simulink model "fec_ber_hw_V2"  (R2020b)
settings: Solver=FixedStepDiscrete  StartTime=0.0  StopTime=T  RelTol=1e-3
values from neighbouring files (symbols this model uses):
  aximm_awgn_reset = 0    [setup.m]
  aximm_bit_count_reset = 0    [setup.m]
  aximm_bits = n_blocks * k    (= 80)    [setup.m]
  aximm_ctrl_word_dec = 0    [setup.m]
  aximm_ctrl_word_enc = 0    [setup.m]
  aximm_enable = 1    [setup.m]
  aximm_length = k * n_blocks    (= 80)    [setup.m]
  aximm_length_dec = n    (= 160)    [setup.m]
  aximm_length_enc = k    (= 80)    [setup.m]
  aximm_llr_mag_reset = 0    [setup.m]
  aximm_llr_scale = (1/noise_var) * llr_scale    (= 1000)    [setup.m]
  aximm_load_dec = 1    [setup.m]
  aximm_load_enc = 1    [setup.m]
  aximm_noise_std = sqrt(noise_var)    [setup.m]
  aximm_reset = 0    [setup.m]
  d = sqrt(-2*log([0:1/4095:1]))    [setup.m]
  fs = 160e6    (= 160000000)    [setup.m]
  generator_polynomial = '''z^13 + z^12 + z^11 + z^8 + 1'''    [setup.m]
  llr_scale = 7.75/7.75    (= 1)    [setup.m]
libraries: simulink x931, hdlsllib x419, commseqgen3 x52, dspsigops x22, commblkcod2 x3, lib_rfsoc_fec x2
(part 2 of 47)

== system fec_ber_hw_V2/Random Number Generator/Random Number Generator ==
  reset : Inport
  enable : EnablePort
  bit0 : commseqgen3/PN Sequence Generator  poly='z^13 + z^12 + z^11 + z^8 + 1'  ini_sta=[ 1 0 1 0 1 0 1 1 0 1 0 0 1]  outBitMaskSource=Dialog parameter  shift=0  outVarSiz=off  maxOutSizeMode=Dialog parameter  maxOutSize=[10 1]  Ts=-1  sampPerFrame=1  reset=on  bitPackedOutputs=off  outDataType=boolean  numPackedBits=8  bitPackDataSigned=off  bitPackedOutDType=double
  bit1 : commseqgen3/PN Sequence Generator  poly='z^13 + z^12 + z^11 + z^8 + 1'  ini_sta=[ 1 0 0 0 0 0 0 0 0 0 0 1 0]  outBitMaskSource=Dialog parameter  shift=0  outVarSiz=off  maxOutSizeMode=Dialog parameter  maxOutSize=[10 1]  Ts=-1  sampPerFrame=1  reset=on  bitPackedOutputs=off  outDataType=boolean  numPackedBits=8  bitPackDataSigned=off  bitPackedOutDType=double
  bit10 : commseqgen3/PN Sequence Generator  poly='z^13 + z^12 + z^11 + z^8 + 1'  ini_sta=[ 0 0 0 0 0 1 0 1 0 0 0 0 1]  outBitMaskSource=Dialog parameter  shift=0  outVarSiz=off  maxOutSizeMode=Dialog parameter  maxOutSize=[10 1]  Ts=-1  sampPerFrame=1  reset=on  bitPackedOutputs=off  outDataType=boolean  numPackedBits=8  bitPackDataSigned=off  bitPackedOutDType=double
  bit11 : commseqgen3/PN Sequence Generator  poly='z^13 + z^12 + z^11 + z^8 + 1'  ini_sta=[ 0 1 1 0 1 1 1 1 0 1 1 0 1]  outBitMaskSource=Dialog parameter  shift=0  outVarSiz=off  maxOutSizeMode=Dialog parameter  maxOutSize=[10 1]  Ts=-1  sampPerFrame=1  reset=on  bitPackedOutputs=off  outDataType=boolean  numPackedBits=8  bitPackDataSigned=off  bitPackedOutDType=double
  bit12 : commseqgen3/PN Sequence Generator  poly='z^13 + z^12 + z^11 + z^8 + 1'  ini_sta=[ 1 1 0 1 0 1 0 1 0 0 0 0 1]  outBitMaskSource=Dialog parameter  shift=0  outVarSiz=off  maxOutSizeMode=Dialog parameter  maxOutSize=[10 1]  Ts=-1  sampPerFrame=1  reset=on  bitPackedOutputs=off  outDataType=boolean  numPackedBits=8  bitPackDataSigned=off  bitPackedOutDType=double
  bit13 : commseqgen3/PN Sequence Generator  poly='z^13 + z^12 + z^11 + z^8 + 1'  ini_sta=[ 1 0 0 1 1 1 1 0 0 0 0 1 0]  outBitMaskSource=Dialog parameter  shift=0  outVarSiz=off  maxOutSizeMode=Dialog parameter  maxOutSize=[10 1]  Ts=-1  sampPerFrame=1  reset=on  bitPackedOutputs=off  outDataType=boolean  numPackedBits=8  bitPackDataSigned=off  bitPackedOutDType=double
  bit14 : commseqgen3/PN Sequence Generator  poly='z^13 + z^12 + z^11 + z^8 + 1'  ini_sta=[ 1 0 0 0 0 1 0 1 0 0 1 0 1]  outBitMaskSource=Dialog parameter  shift=0  outVarSiz=off  maxOutSizeMode=Dialog parameter  maxOutSize=[10 1]  Ts=-1  sampPerFrame=1  reset=on  bitPackedOutputs=off  outDataType=boolean  numPackedBits=8  bitPackDataSigned=off  bitPackedOutDType=double
  bit15 : commseqgen3/PN Sequence Generator  poly='z^13 + z^12 + z^11 + z^8 + 1'  ini_sta=[ 1 1 0 1 1 1 0 1 0 0 1 0 0]  outBitMaskSource=Dialog parameter  shift=0  outVarSiz=off  maxOutSizeMode=Dialog parameter  maxOutSize=[10 1]  Ts=-1  sampPerFrame=1  reset=on  bitPackedOutputs=off  outDataType=boolean  numPackedBits=8  bitPackDataSigned=off  bitPackedOutDType=double
  bit16 : commseqgen3/PN Sequence Generator  poly='z^13 + z^12 + z^11 + z^8 + 1'  ini_sta=[ 0 0 0 1 1 0 0 1 0 0 0 0 1]  outBitMaskSource=Dialog parameter  shift=0  outVarSiz=off  maxOutSizeMode=Dialog parameter  maxOutSize=[10 1]  Ts=-1  sampPerFrame=1  reset=on  bitPackedOutputs=off  outDataType=boolean  numPackedBits=8  bitPackDataSigned=off  bitPackedOutDType=double
  bit17 : commseqgen3/PN Sequence Generator  poly='z^13 + z^12 + z^11 + z^8 + 1'  ini_sta=[ 1 1 1 0 1 0 0 0 0 1 1 1 0]  outBitMaskSource=Dialog parameter  shift=0  outVarSiz=off  maxOutSizeMode=Dialog parameter  maxOutSize=[10 1]  Ts=-1  sampPerFrame=1  reset=on  bitPackedOutputs=off  outDataType=boolean  numPackedBits=8  bitPackDataSigned=off  bitPackedOutDType=double
  bit18 : commseqgen3/PN Sequence Generator  poly='z^13 + z^12 + z^11 + z^8 + 1'  ini_sta=[ 0 0 0 1 1 0 1 1 1 0 1 0 1]  outBitMaskSource=Dialog parameter  shift=0  outVarSiz=off  maxOutSizeMode=Dialog parameter  maxOutSize=[10 1]  Ts=-1  sampPerFrame=1  reset=on  bitPackedOutputs=off  outDataType=boolean  numPackedBits=8  bitPackDataSigned=off  bitPackedOutDType=double
  bit19 : commseqgen3/PN Sequence Generator  poly='z^13 + z^12 + z^11 + z^8 + 1'  ini_sta=[ 1 0 0 0 0 1 0 0 0 1 0 1 1]  outBitMaskSource=Dialog parameter  shift=0  outVarSiz=off  maxOutSizeMode=Dialog parameter  maxOutSize=[10 1]  Ts=-1  sampPerFrame=1  reset=on  bitPackedOutputs=off  outDataType=boolean  numPackedBits=8  bitPackDataSigned=off  bitPackedOutDType=double
  bit2 : commseqgen3/PN Sequence Generator  poly='z^13 + z^12 + z^11 + z^8 + 1'  ini_sta=[ 0 0 1 1 0 1 1 1 1 1 0 1 0]  outBitMaskSource=Dialog parameter  shift=0  outVarSiz=off  maxOutSizeMode=Dialog parameter  maxOutSize=[10 1]  Ts=-1  sampPerFrame=1  reset=on  bitPackedOutputs=off  outDataType=boolean  numPackedBits=8  bitPackDataSigned=off  bitPackedOutDType=double
  bit20 : commseqgen3/PN Sequence Generator  poly='z^13 + z^12 + z^11 + z^8 + 1'  ini_sta=[ 0 0 1 0 0 1 0 0 1 0 1 0 1]  outBitMaskSource=Dialog parameter  shift=0  outVarSiz=off  maxOutSizeMode=Dialog parameter  maxOutSize=[10 1]  Ts=-1  sampPerFrame=1  reset=on  bitPackedOutputs=off  outDataType=boolean  numPackedBits=8  bitPackDataSigned=off  bitPackedOutDType=double
  bit21 : commseqgen3/PN Sequence Generator  poly='z^13 + z^12 + z^11 + z^8 + 1'  ini_sta=[ 1 0 0 0 1 1 1 1 0 0 1 1 0]  outBitMaskSource=Dialog parameter  shift=0  outVarSiz=off  maxOutSizeMode=Dialog parameter  maxOutSize=[10 1]  Ts=-1  sampPerFrame=1  reset=on  bitPackedOutputs=off  outDataType=boolean  numPackedBits=8  bitPackDataSigned=off  bitPackedOutDType=double
  bit22 : commseqgen3/PN Sequence Generator  poly='z^13 + z^12 + z^11 + z^8 + 1'  ini_sta=[ 0 0 0 0 0 0 0 1 0 0 1 1 0]  outBitMaskSource=Dialog parameter  shift=0  outVarSiz=off  maxOutSizeMode=Dialog parameter  maxOutSize=[10 1]  Ts=-1  sampPerFrame=1  reset=on  bitPackedOutputs=off  outDataType=boolean  numPackedBits=8  bitPackDataSigned=off  bitPackedOutDType=double
  bit23 : commseqgen3/PN Sequence Generator  poly='z^13 + z^12 + z^11 + z^8 + 1'  ini_sta=[ 1 1 0 0 0 1 0 0 0 1 0 0 0]  outBitMaskSource=Dialog parameter  shift=0  outVarSiz=off  maxOutSizeMode=Dialog parameter  maxOutSize=[10 1]  Ts=-1  sampPerFrame=1  reset=on  bitPackedOutputs=off  outDataType=boolean  numPackedBits=8  bitPackDataSigned=off  bitPackedOutDType=double
  bit24 : commseqgen3/PN Sequence Generator  poly='z^13 + z^12 + z^11 + z^8 + 1'  ini_sta=[ 1 1 0 1 1 0 0 1 0 1 0 0 0]  outBitMaskSource=Dialog parameter  shift=0  outVarSiz=off  maxOutSizeMode=Dialog parameter  maxOutSize=[10 1]  Ts=-1  sampPerFrame=1  reset=on  bitPackedOutputs=off  outDataType=boolean  numPackedBits=8  bitPackDataSigned=off  bitPackedOutDType=double
  bit25 : commseqgen3/PN Sequence Generator  poly='z^13 + z^12 + z^11 + z^8 + 1'  ini_sta=[ 1 1 1 0 1 0 1 0 1 0 1 1 0]  outBitMaskSource=Dialog parameter  shift=0  outVarSiz=off  maxOutSizeMode=Dialog parameter  maxOutSize=[10 1]  Ts=-1  sampPerFrame=1  reset=on  bitPackedOutputs=off  outDataType=boolean  numPackedBits=8  bitPackDataSigned=off  bitPackedOutDType=double
  bit26 : commseqgen3/PN Sequence Generator  poly='z^13 + z^12 + z^11 + z^8 + 1'  ini_sta=[ 1 1 1 1 1 1 0 0 1 0 1 0 1]  outBitMaskSource=Dialog parameter  shift=0  outVarSiz=off  maxOutSizeMode=Dialog parameter  maxOutSize=[10 1]  Ts=-1  sampPerFrame=1  reset=on  bitPackedOutputs=off  outDataType=boolean  numPackedBits=8  bitPackDataSigned=off  bitPackedOutDType=double
  bit27 : commseqgen3/PN Sequence Generator  poly='z^13 + z^12 + z^11 + z^8 + 1'  ini_sta=[ 1 0 0 0 0 0 0 1 0 1 0 1 0]  outBitMaskSource=Dialog parameter  shift=0  outVarSiz=off  maxOutSizeMode=Dialog parameter  maxOutSize=[10 1]  Ts=-1  sampPerFrame=1  reset=on  bitPackedOutputs=off  outDataType=boolean  numPackedBits=8  bitPackDataSigned=off  bitPackedOutDType=double
  bit28 : commseqgen3/PN Sequence Generator  poly='z^13 + z^12 + z^11 + z^8 + 1'  ini_sta=[ 0 1 0 0 0 1 0 1 1 0 0 0 0]  outBitMaskSource=Dialog parameter  shift=0  outVarSiz=off  maxOutSizeMode=Dialog parameter  maxOutSize=[10 1]  Ts=-1  sampPerFrame=1  reset=on  bitPackedOutputs=off  outDataType=boolean  numPackedBits=8  bitPackDataSigned=off  bitPackedOutDType=double
  bit29 : commseqgen3/PN Sequence Generator  poly='z^13 + z^12 + z^11 + z^8 + 1'  ini_sta=[ 0 0 0 1 1 0 0 1 1 1 0 1 0]  outBitMaskSource=Dialog parameter  shift=0  outVarSiz=off  maxOutSizeMode=Dialog parameter  maxOutSize=[10 1]  Ts=-1  sampPerFrame=1  reset=on  bitPackedOutputs=off  outDataType=boolean  numPackedBits=8  bitPackDataSigned=off  bitPackedOutDType=double
  bit3 : commseqgen3/PN Sequence Generator  poly='z^13 + z^12 + z^11 + z^8 + 1'  ini_sta=[ 1 0 0 1 0 0 1 0 0 1 0 1 1]  outBitMaskSource=Dialog parameter  shift=0  outVarSiz=off  maxOutSizeMode=Dialog parameter  maxOutSize=[10 1]  Ts=-1  sampPerFrame=1  reset=on  bitPackedOutputs=off  outDataType=boolean  numPackedBits=8  bitPackDataSigned=off  bitPackedOutDType=double
  bit30 : commseqgen3/PN Sequence Generator  poly='z^13 + z^12 + z^11 + z^8 + 1'  ini_sta=[ 1 0 0 0 0 0 1 0 0 0 0 0 0]  outBitMaskSource=Dialog parameter  shift=0  outVarSiz=off  maxOutSizeMode=Dialog parameter  maxOutSize=[10 1]  Ts=-1  sampPerFrame=1  reset=on  bitPackedOutputs=off  outDataType=boolean  numPackedBits=8  bitPackDataSigned=off  bitPackedOutDType=double
  bit31 : commseqgen3/PN Sequence Generator  poly='z^13 + z^12 + z^11 + z^8 + 1'  ini_sta=[ 1 0 0 1 0 1 0 1 1 1 1 0 1]  outBitMaskSource=Dialog parameter  shift=0  outVarSiz=off  maxOutSizeMode=Dialog parameter  maxOutSize=[10 1]  Ts=-1  sampPerFrame=1  reset=on  bitPackedOutputs=off  outDataType=boolean  numPackedBits=8  bitPackDataSigned=off  bitPackedOutDType=double
  bit4 : commseqgen3/PN Sequence Generator  poly='z^13 + z^12 + z^11 + z^8 + 1'  ini_sta=[ 0 0 0 1 1 1 1 1 0 1 0 0 1]  outBitMaskSource=Dialog parameter  shift=0  outVarSiz=off  maxOutSizeMode=Dialog parameter  maxOutSize=[10 1]  Ts=-1  sampPerFrame=1  reset=on  bitPackedOutputs=off  outDataType=boolean  numPackedBits=8  bitPackDataSigned=off  bitPackedOutDType=double
  bit5 : commseqgen3/PN Sequence Generator  poly='z^13 + z^12 + z^11 + z^8 + 1'  ini_sta=[ 1 0 1 0 1 0 1 1 1 1 0 1 0]  outBitMaskSource=Dialog parameter  shift=0  outVarSiz=off  maxOutSizeMode=Dialog parameter  maxOutSize=[10 1]  Ts=-1  sampPerFrame=1  reset=on  bitPackedOutputs=off  outDataType=boolean  numPackedBits=8  bitPackDataSigned=off  bitPackedOutDType=double
  bit6 : commseqgen3/PN Sequence Generator  poly='z^13 + z^12 + z^11 + z^8 + 1'  ini_sta=[ 1 0 0 1 1 0 0 1 1 0 0 0 0]  outBitMaskSource=Dialog parameter  shift=0  outVarSiz=off  maxOutSizeMode=Dialog parameter  maxOutSize=[10 1]  Ts=-1  sampPerFrame=1  reset=on  bitPackedOutputs=off  outDataType=boolean  numPackedBits=8  bitPackDataSigned=off  bitPackedOutDType=double
  bit7 : commseqgen3/PN Sequence Generator  poly='z^13 + z^12 + z^11 + z^8 + 1'  ini_sta=[ 0 0 0 0 1 1 1 0 0 1 0 1 1]  outBitMaskSource=Dialog parameter  shift=0  outVarSiz=off  maxOutSizeMode=Dialog parameter  maxOutSize=[10 1]  Ts=-1  sampPerFrame=1  reset=on  bitPackedOutputs=off  outDataType=boolean  numPackedBits=8  bitPackDataSigned=off  bitPackedOutDType=double
  bit8 : commseqgen3/PN Sequence Generator  poly='z^13 + z^12 + z^11 + z^8 + 1'  ini_sta=[ 0 0 0 0 1 1 1 0 0 1 1 1 0]  outBitMaskSource=Dialog parameter  shift=0  outVarSiz=off  maxOutSizeMode=Dialog parameter  maxOutSize=[10 1]  Ts=-1  sampPerFrame=1  reset=on  bitPackedOutputs=off  outDataType=boolean  numPackedBits=8  bitPackDataSigned=off  bitPackedOutDType=double
  bit9 : commseqgen3/PN Sequence Generator  poly='z^13 + z^12 + z^11 + z^8 + 1'  ini_sta=[ 0 0 1 0 0 1 1 1 0 0 0 1 0]  outBitMaskSource=Dialog parameter  shift=0  outVarSiz=off  maxOutSizeMode=Dialog parameter  maxOutSize=[10 1]  Ts=-1  sampPerFrame=1  reset=on  bitPackedOutputs=off  outDataType=boolean  numPackedBits=8  bitPackDataSigned=off  bitPackedOutDType=double
  concat : hdlsllib/Logic and Bit Operations/Bit Concat  numInputs=32
  data : Outport
  wires:
  reset/1 -> bit0/1, bit1/1, bit2/1, bit3/1, bit4/1, bit5/1, bit6/1, bit7/1, bit8/1, bit9/1, bit10/1, bit11/1, bit12/1, bit13/1, bit14/1, bit15/1, bit16/1, bit17/1, bit18/1, bit19/1, bit20/1, bit21/1, bit22/1, bit23/1, bit24/1, bit25/1, bit26/1, bit27/1, bit28/1, bit29/1, bit30/1, bit31/1
  bit0/1 -> concat/1
  bit1/1 -> concat/2
  bit2/1 -> concat/3
  bit3/1 -> concat/4
  bit4/1 -> concat/5
  bit5/1 -> concat/6
  bit6/1 -> concat/7
  bit7/1 -> concat/8
  bit8/1 -> concat/9
  bit9/1 -> concat/10
  bit10/1 -> concat/11
  bit11/1 -> concat/12
  bit12/1 -> concat/13
  bit13/1 -> concat/14
  bit14/1 -> concat/15
  bit15/1 -> concat/16
  bit16/1 -> concat/17
  bit17/1 -> concat/18
  bit18/1 -> concat/19
  bit19/1 -> concat/20
  bit20/1 -> concat/21
  bit21/1 -> concat/22
  bit22/1 -> concat/23
  bit23/1 -> concat/24
  bit24/1 -> concat/25
  bit25/1 -> concat/26
  bit26/1 -> concat/27
  bit27/1 -> concat/28
  bit28/1 -> concat/29
  bit29/1 -> concat/30
  bit30/1 -> concat/31
  bit31/1 -> concat/32
  concat/1 -> data/1

== system fec_ber_hw_V2/Random Number Generator/concat ==
  en : Inport
  diff : Inport  Port=2
  d_in : Inport  Port=3
  Bitwise Operator : simulink/Logic and Bit Operations/Bitwise Operator  logicop=AND  UseBitMask=off  NumInputPorts=2  BitMask=bin2dec('11011001')  BitMaskRealWorld=Stored Integer
  Constant : Constant  Value=0  OutDataTypeStr=fixdt(0,32,0)  SampleTime=-1
  Delay : Delay  DelayLength=1
  Delay1 : Delay  DelayLength=1
  Multiport Switch : MultiPortSwitch  DataPortOrder=Zero-based contiguous  Inputs=2  zeroidx=on
  mask_generator : Subsystem
  d_out : Outport
  wires:
  d_in/1 -> Delay1/1
  diff/1 -> mask_generator/1(diff)
  Delay1/1 -> Bitwise Operator/1
  mask_generator/1(mask) -> Bitwise Operator/2
  Multiport Switch/1 -> d_out/1
  en/1 -> Delay/1, mask_generator/2(sel)
  Bitwise Operator/1 -> Multiport Switch/3
  Constant/1 -> Multiport Switch/2
  Delay/1 -> Multiport Switch/1

== system fec_ber_hw_V2/Random Number Generator/rising_edge ==
  in : Inport
  Data Type Conversion1 : DataTypeConversion  OutDataTypeStr=boolean  SaturateOnIntegerOverflow=on  RndMeth=Zero
  Delay15 : Delay  DelayLength=1  InitialCondition=1  InputProcessing=Columns as channels (frame based)
  Logical Operator2 : Logic  Operator=NOT  Inputs=1
  Logical Operator3 : Logic
  pulse : Outport
  wires:
  Delay15/1 -> Logical Operator2/1
  Logical Operator3/1 -> pulse/1
  Data Type Conversion1/1 -> Delay15/1, Logical Operator3/1
  in/1 -> Data Type Conversion1/1
  Logical Operator2/1 -> Logical Operator3/2

== system fec_ber_hw_V2/Random Number Generator/tvalid hold ==
  trigger : Inport
  comparator : Inport  Port=2
  Delay2 : Delay  DelayLength=1
  Equal : RelationalOperator  OutDataTypeStr=boolean  RndMeth=Simplest
  HDL Counter : hdlsllib/Sources/HDL Counter  CountType=Free running  CountInit=0  CountStep=32  CountMax=25  CountFromType=Initial value  CountFrom=0  CountResetPort=on  CountLoadPort=off  CountEnbPort=on  CountDirPort=off  CountDataType=Unsigned  CountWordLen=32  CountFracLen=0  CountSampTime=1
  Multiport Switch : MultiPortSwitch  DataPortOrder=Zero-based contiguous  Inputs=2  zeroidx=on
  OR : Logic  Operator=OR  IconShape=distinctive  AllPortsSameDT=off  OutDataTypeStr=boolean
  Subtract : Sum  Inputs=+-
  enable : Outport
  diff : Outport  Port=2
  wires:
  OR/1 -> Multiport Switch/1
  Delay2/1 -> Multiport Switch/2
  comparator/1 -> Subtract/2, Equal/2
  trigger/1 -> OR/2, Multiport Switch/3
  Equal/1 -> OR/1, HDL Counter/1
  HDL Counter/1 -> Subtract/1, Equal/1
  Subtract/1 -> diff/1
  Multiport Switch/1 -> HDL Counter/2, enable/1, Delay2/1

== system fec_ber_hw_V2/Soft Demodulation/SSR Soft Demodulation Lane 0 ==
  valid : Inport
  real : Inport  Port=2
  imag : Inport  Port=3
  scale : Inport  Port=4
  Soft Demodulation 0 : Subsystem  mask{w=3, f=0, n=1}
  Soft Demodulation 1 : Subsystem  mask{w=3, f=0, n=7}
  Soft Demodulation 2 : Subsystem  mask{w=3, f=0, n=6}
  Soft Demodulation 3 : Subsystem  mask{w=3, f=0, n=5}
  Soft Demodulation 4 : Subsystem  mask{w=3, f=0, n=4}
  Soft Demodulation 5 : Subsystem  mask{w=3, f=0, n=3}
  Soft Demodulation 6 : Subsystem  mask{w=3, f=0, n=2}
  Soft Demodulation 7 : Subsystem  mask{w=3, f=0, n=1}
  concat : hdlsllib/Logic and Bit Operations/Bit Concat  numInputs=8
  llr : Outport
  wires:
  valid/1 -> Soft Demodulation 0/1(valid), Soft Demodulation 1/1(valid), Soft Demodulation 2/1(valid), Soft Demodulation 3/1(valid), Soft Demodulation 4/1(valid), Soft Demodulation 5/1(valid), Soft Demodulation 6/1(valid), Soft Demodulation 7/1(valid)
  real/1 -> Soft Demodulation 0/2(real), Soft Demodulation 1/2(real), Soft Demodulation 2/2(real), Soft Demodulation 3/2(real), Soft Demodulation 4/2(real), Soft Demodulation 5/2(real), Soft Demodulation 6/2(real), Soft Demodulation 7/2(real)
  imag/1 -> Soft Demodulation 0/3(imag), Soft Demodulation 1/3(imag), Soft Demodulation 2/3(imag), Soft Demodulation 3/3(imag), Soft Demodulation 4/3(imag), Soft Demodulation 5/3(imag), Soft Demodulation 6/3(imag), Soft Demodulation 7/3(imag)
  scale/1 -> Soft Demodulation 0/4(LLR Scale), Soft Demodulation 1/4(LLR Scale), Soft Demodulation 2/4(LLR Scale), Soft Demodulation 3/4(LLR Scale), Soft Demodulation 4/4(LLR Scale), Soft Demodulation 5/4(LLR Scale), Soft Demodulation 6/4(LLR Scale), Soft Demodulation 7/4(LLR Scale)
  Soft Demodulation 0/1(LLR Values) -> concat/1
  Soft Demodulation 1/1(LLR Values) -> concat/2
  Soft Demodulation 2/1(LLR Values) -> concat/3
  Soft Demodulation 3/1(LLR Values) -> concat/4
  Soft Demodulation 4/1(LLR Values) -> concat/5
  Soft Demodulation 5/1(LLR Values) -> concat/6
  Soft Demodulation 6/1(LLR Values) -> concat/7
  Soft Demodulation 7/1(LLR Values) -> concat/8
  concat/1 -> llr/1

== system fec_ber_hw_V2/Soft Demodulation/SSR Soft Demodulation Lane 1 ==
  valid : Inport
  real : Inport  Port=2
  imag : Inport  Port=3
  scale : Inport  Port=4
  Soft Demodulation 0 : Subsystem  mask{w=3, f=0, n=16}
  Soft Demodulation 1 : Subsystem  mask{w=3, f=0, n=15}
  Soft Demodulation 10 : Subsystem  mask{w=3, f=0, n=6}
  Soft Demodulation 11 : Subsystem  mask{w=3, f=0, n=5}
  Soft Demodulation 12 : Subsystem  mask{w=3, f=0, n=4}
  Soft Demodulation 13 : Subsystem  mask{w=3, f=0, n=3}
  Soft Demodulation 14 : Subsystem  mask{w=3, f=0, n=2}
  Soft Demodulation 15 : Subsystem  mask{w=3, f=0, n=1}
  Soft Demodulation 2 : Subsystem  mask{w=3, f=0, n=14}
  Soft Demodulation 3 : Subsystem  mask{w=3, f=0, n=13}
  Soft Demodulation 4 : Subsystem  mask{w=3, f=0, n=12}
  Soft Demodulation 5 : Subsystem  mask{w=3, f=0, n=11}
  Soft Demodulation 6 : Subsystem  mask{w=3, f=0, n=10}
  Soft Demodulation 7 : Subsystem  mask{w=3, f=0, n=9}
  Soft Demodulation 8 : Subsystem  mask{w=3, f=0, n=8}
  Soft Demodulation 9 : Subsystem  mask{w=3, f=0, n=7}
  concat : hdlsllib/Logic and Bit Operations/Bit Concat  numInputs=16
  llr : Outport
  wires:
  valid/1 -> Soft Demodulation 0/1(valid), Soft Demodulation 1/1(valid), Soft Demodulation 2/1(valid), Soft Demodulation 3/1(valid), Soft Demodulation 4/1(valid), Soft Demodulation 5/1(valid), Soft Demodulation 6/1(valid), Soft Demodulation 7/1(valid), Soft Demodulation 8/1(valid), Soft Demodulation 9/1(valid), Soft Demodulation 10/1(valid), Soft Demodulation 11/1(valid), Soft Demodulation 12/1(valid), Soft Demodulation 13/1(valid), Soft Demodulation 14/1(valid), Soft Demodulation 15/1(valid)
  real/1 -> Soft Demodulation 0/2(real), Soft Demodulation 1/2(real), Soft Demodulation 2/2(real), Soft Demodulation 3/2(real), Soft Demodulation 4/2(real), Soft Demodulation 5/2(real), Soft Demodulation 6/2(real), Soft Demodulation 7/2(real), Soft Demodulation 8/2(real), Soft Demodulation 9/2(real), Soft Demodulation 10/2(real), Soft Demodulation 11/2(real), Soft Demodulation 12/2(real), Soft Demodulation 13/2(real), Soft Demodulation 14/2(real), Soft Demodulation 15/2(real)
  imag/1 -> Soft Demodulation 0/3(imag), Soft Demodulation 1/3(imag), Soft Demodulation 2/3(imag), Soft Demodulation 3/3(imag), Soft Demodulation 4/3(imag), Soft Demodulation 5/3(imag), Soft Demodulation 6/3(imag), Soft Demodulation 7/3(imag), Soft Demodulation 8/3(imag), Soft Demodulation 9/3(imag), Soft Demodulation 10/3(imag), Soft Demodulation 11/3(imag), Soft Demodulation 12/3(imag), Soft Demodulation 13/3(imag), Soft Demodulation 14/3(imag), Soft Demodulation 15/3(imag)
  scale/1 -> Soft Demodulation 0/4(LLR Scale), Soft Demodulation 1/4(LLR Scale), Soft Demodulation 2/4(LLR Scale), Soft Demodulation 3/4(LLR Scale), Soft Demodulation 4/4(LLR Scale), Soft Demodulation 5/4(LLR Scale), Soft Demodulation 6/4(LLR Scale), Soft Demodulation 7/4(LLR Scale), Soft Demodulation 8/4(LLR Scale), Soft Demodulation 9/4(LLR Scale), Soft Demodulation 10/4(LLR Scale), Soft Demodulation 11/4(LLR Scale), Soft Demodulation 12/4(LLR Scale), Soft Demodulation 13/4(LLR Scale), Soft Demodulation 14/4(LLR Scale), Soft Demodulation 15/4(LLR Scale)
  Soft Demodulation 0/1(LLR Values) -> concat/1
  Soft Demodulation 1/1(LLR Values) -> concat/2
  Soft Demodulation 2/1(LLR Values) -> concat/3
  Soft Demodulation 3/1(LLR Values) -> concat/4
  Soft Demodulation 4/1(LLR Values) -> concat/5
  Soft Demodulation 5/1(LLR Values) -> concat/6
  Soft Demodulation 6/1(LLR Values) -> concat/7
  Soft Demodulation 7/1(LLR Values) -> concat/8
  Soft Demodulation 8/1(LLR Values) -> concat/9
  Soft Demodulation 9/1(LLR Values) -> concat/10
  Soft Demodulation 10/1(LLR Values) -> concat/11
  Soft Demodulation 11/1(LLR Values) -> concat/12
  Soft Demodulation 12/1(LLR Values) -> concat/13
  Soft Demodulation 13/1(LLR Values) -> concat/14
  Soft Demodulation 14/1(LLR Values) -> concat/15
  Soft Demodulation 15/1(LLR Values) -> concat/16
  concat/1 -> llr/1

== system fec_ber_hw_V2/Soft Demodulation/SSR Soft Demodulation Lane 2 ==
  valid : Inport
  real : Inport  Port=2
  imag : Inport  Port=3
  scale : Inport  Port=4
  Soft Demodulation 0 : Subsystem  mask{w=3, f=0, n=16}
  Soft Demodulation 1 : Subsystem  mask{w=3, f=0, n=15}
  Soft Demodulation 10 : Subsystem  mask{w=3, f=0, n=6}
  Soft Demodulation 11 : Subsystem  mask{w=3, f=0, n=5}
  Soft Demodulation 12 : Subsystem  mask{w=3, f=0, n=4}
  Soft Demodulation 13 : Subsystem  mask{w=3, f=0, n=3}
  Soft Demodulation 14 : Subsystem  mask{w=3, f=0, n=2}
  Soft Demodulation 15 : Subsystem  mask{w=3, f=0, n=1}
  Soft Demodulation 2 : Subsystem  mask{w=3, f=0, n=14}
  Soft Demodulation 3 : Subsystem  mask{w=3, f=0, n=13}
  Soft Demodulation 4 : Subsystem  mask{w=3, f=0, n=12}
  Soft Demodulation 5 : Subsystem  mask{w=3, f=0, n=11}
  Soft Demodulation 6 : Subsystem  mask{w=3, f=0, n=10}
  Soft Demodulation 7 : Subsystem  mask{w=3, f=0, n=9}
  Soft Demodulation 8 : Subsystem  mask{w=3, f=0, n=8}
  Soft Demodulation 9 : Subsystem  mask{w=3, f=0, n=7}
  concat : hdlsllib/Logic and Bit Operations/Bit Concat  numInputs=16
  llr : Outport
  wires:
  valid/1 -> Soft Demodulation 0/1(valid), Soft Demodulation 1/1(valid), Soft Demodulation 2/1(valid), Soft Demodulation 3/1(valid), Soft Demodulation 4/1(valid), Soft Demodulation 5/1(valid), Soft Demodulation 6/1(valid), Soft Demodulation 7/1(valid), Soft Demodulation 8/1(valid), Soft Demodulation 9/1(valid), Soft Demodulation 10/1(valid), Soft Demodulation 11/1(valid), Soft Demodulation 12/1(valid), Soft Demodulation 13/1(valid), Soft Demodulation 14/1(valid), Soft Demodulation 15/1(valid)
  real/1 -> Soft Demodulation 0/2(real), Soft Demodulation 1/2(real), Soft Demodulation 2/2(real), Soft Demodulation 3/2(real), Soft Demodulation 4/2(real), Soft Demodulation 5/2(real), Soft Demodulation 6/2(real), Soft Demodulation 7/2(real), Soft Demodulation 8/2(real), Soft Demodulation 9/2(real), Soft Demodulation 10/2(real), Soft Demodulation 11/2(real), Soft Demodulation 12/2(real), Soft Demodulation 13/2(real), Soft Demodulation 14/2(real), Soft Demodulation 15/2(real)
  imag/1 -> Soft Demodulation 0/3(imag), Soft Demodulation 1/3(imag), Soft Demodulation 2/3(imag), Soft Demodulation 3/3(imag), Soft Demodulation 4/3(imag), Soft Demodulation 5/3(imag), Soft Demodulation 6/3(imag), Soft Demodulation 7/3(imag), Soft Demodulation 8/3(imag), Soft Demodulation 9/3(imag), Soft Demodulation 10/3(imag), Soft Demodulation 11/3(imag), Soft Demodulation 12/3(imag), Soft Demodulation 13/3(imag), Soft Demodulation 14/3(imag), Soft Demodulation 15/3(imag)
  scale/1 -> Soft Demodulation 0/4(LLR Scale), Soft Demodulation 1/4(LLR Scale), Soft Demodulation 2/4(LLR Scale), Soft Demodulation 3/4(LLR Scale), Soft Demodulation 4/4(LLR Scale), Soft Demodulation 5/4(LLR Scale), Soft Demodulation 6/4(LLR Scale), Soft Demodulation 7/4(LLR Scale), Soft Demodulation 8/4(LLR Scale), Soft Demodulation 9/4(LLR Scale), Soft Demodulation 10/4(LLR Scale), Soft Demodulation 11/4(LLR Scale), Soft Demodulation 12/4(LLR Scale), Soft Demodulation 13/4(LLR Scale), Soft Demodulation 14/4(LLR Scale), Soft Demodulation 15/4(LLR Scale)
  Soft Demodulation 0/1(LLR Values) -> concat/1
  Soft Demodulation 1/1(LLR Values) -> concat/2
  Soft Demodulation 2/1(LLR Values) -> concat/3
  Soft Demodulation 3/1(LLR Values) -> concat/4
  Soft Demodulation 4/1(LLR Values) -> concat/5
  Soft Demodulation 5/1(LLR Values) -> concat/6
  Soft Demodulation 6/1(LLR Values) -> concat/7
  Soft Demodulation 7/1(LLR Values) -> concat/8
  Soft Demodulation 8/1(LLR Values) -> concat/9
  Soft Demodulation 9/1(LLR Values) -> concat/10
  Soft Demodulation 10/1(LLR Values) -> concat/11
  Soft Demodulation 11/1(LLR Values) -> concat/12
  Soft Demodulation 12/1(LLR Values) -> concat/13
  Soft Demodulation 13/1(LLR Values) -> concat/14
  Soft Demodulation 14/1(LLR Values) -> concat/15
  Soft Demodulation 15/1(LLR Values) -> concat/16
  concat/1 -> llr/1

== system fec_ber_hw_V2/Soft Demodulation/SSR Soft Demodulation Lane 3 ==
  valid : Inport
  real : Inport  Port=2
  imag : Inport  Port=3
  scale : Inport  Port=4
  Soft Demodulation 0 : Subsystem  mask{w=3, f=0, n=16}
  Soft Demodulation 1 : Subsystem  mask{w=3, f=0, n=15}
  Soft Demodulation 10 : Subsystem  mask{w=3, f=0, n=6}
  Soft Demodulation 11 : Subsystem  mask{w=3, f=0, n=5}
  Soft Demodulation 12 : Subsystem  mask{w=3, f=0, n=4}
  Soft Demodulation 13 : Subsystem  mask{w=3, f=0, n=3}
  Soft Demodulation 14 : Subsystem  mask{w=3, f=0, n=2}
  Soft Demodulation 15 : Subsystem  mask{w=3, f=0, n=1}
  Soft Demodulation 2 : Subsystem  mask{w=3, f=0, n=14}
  Soft Demodulation 3 : Subsystem  mask{w=3, f=0, n=13}
  Soft Demodulation 4 : Subsystem  mask{w=3, f=0, n=12}
  Soft Demodulation 5 : Subsystem  mask{w=3, f=0, n=11}
  Soft Demodulation 6 : Subsystem  mask{w=3, f=0, n=10}
  Soft Demodulation 7 : Subsystem  mask{w=3, f=0, n=9}
  Soft Demodulation 8 : Subsystem  mask{w=3, f=0, n=8}
  Soft Demodulation 9 : Subsystem  mask{w=3, f=0, n=7}
  concat : hdlsllib/Logic and Bit Operations/Bit Concat  numInputs=16
  llr : Outport
  wires:
  valid/1 -> Soft Demodulation 0/1(valid), Soft Demodulation 1/1(valid), Soft Demodulation 2/1(valid), Soft Demodulation 3/1(valid), Soft Demodulation 4/1(valid), Soft Demodulation 5/1(valid), Soft Demodulation 6/1(valid), Soft Demodulation 7/1(valid), Soft Demodulation 8/1(valid), Soft Demodulation 9/1(valid), Soft Demodulation 10/1(valid), Soft Demodulation 11/1(valid), Soft Demodulation 12/1(valid), Soft Demodulation 13/1(valid), Soft Demodulation 14/1(valid), Soft Demodulation 15/1(valid)
  real/1 -> Soft Demodulation 0/2(real), Soft Demodulation 1/2(real), Soft Demodulation 2/2(real), Soft Demodulation 3/2(real), Soft Demodulation 4/2(real), Soft Demodulation 5/2(real), Soft Demodulation 6/2(real), Soft Demodulation 7/2(real), Soft Demodulation 8/2(real), Soft Demodulation 9/2(real), Soft Demodulation 10/2(real), Soft Demodulation 11/2(real), Soft Demodulation 12/2(real), Soft Demodulation 13/2(real), Soft Demodulation 14/2(real), Soft Demodulation 15/2(real)
  imag/1 -> Soft Demodulation 0/3(imag), Soft Demodulation 1/3(imag), Soft Demodulation 2/3(imag), Soft Demodulation 3/3(imag), Soft Demodulation 4/3(imag), Soft Demodulation 5/3(imag), Soft Demodulation 6/3(imag), Soft Demodulation 7/3(imag), Soft Demodulation 8/3(imag), Soft Demodulation 9/3(imag), Soft Demodulation 10/3(imag), Soft Demodulation 11/3(imag), Soft Demodulation 12/3(imag), Soft Demodulation 13/3(imag), Soft Demodulation 14/3(imag), Soft Demodulation 15/3(imag)
  scale/1 -> Soft Demodulation 0/4(LLR Scale), Soft Demodulation 1/4(LLR Scale), Soft Demodulation 2/4(LLR Scale), Soft Demodulation 3/4(LLR Scale), Soft Demodulation 4/4(LLR Scale), Soft Demodulation 5/4(LLR Scale), Soft Demodulation 6/4(LLR Scale), Soft Demodulation 7/4(LLR Scale), Soft Demodulation 8/4(LLR Scale), Soft Demodulation 9/4(LLR Scale), Soft Demodulation 10/4(LLR Scale), Soft Demodulation 11/4(LLR Scale), Soft Demodulation 12/4(LLR Scale), Soft Demodulation 13/4(LLR Scale), Soft Demodulation 14/4(LLR Scale), Soft Demodulation 15/4(LLR Scale)
  Soft Demodulation 0/1(LLR Values) -> concat/1
  Soft Demodulation 1/1(LLR Values) -> concat/2
  Soft Demodulation 2/1(LLR Values) -> concat/3
  Soft Demodulation 3/1(LLR Values) -> concat/4
  Soft Demodulation 4/1(LLR Values) -> concat/5
  Soft Demodulation 5/1(LLR Values) -> concat/6
  Soft Demodulation 6/1(LLR Values) -> concat/7
  Soft Demodulation 7/1(LLR Values) -> concat/8
  Soft Demodulation 8/1(LLR Values) -> concat/9
  Soft Demodulation 9/1(LLR Values) -> concat/10
  Soft Demodulation 10/1(LLR Values) -> concat/11
  Soft Demodulation 11/1(LLR Values) -> concat/12
  Soft Demodulation 12/1(LLR Values) -> concat/13
  Soft Demodulation 13/1(LLR Values) -> concat/14
  Soft Demodulation 14/1(LLR Values) -> concat/15
  Soft Demodulation 15/1(LLR Values) -> concat/16
  concat/1 -> llr/1

== system fec_ber_hw_V2/Soft Demodulation/SSR Soft Demodulation Lane 4 ==
  valid : Inport
  real : Inport  Port=2
  imag : Inport  Port=3
  scale : Inport  Port=4
  Soft Demodulation 0 : Subsystem  mask{w=3, f=0, n=1}
  Soft Demodulation 1 : Subsystem  mask{w=3, f=0, n=7}
  Soft Demodulation 2 : Subsystem  mask{w=3, f=0, n=6}
  Soft Demodulation 3 : Subsystem  mask{w=3, f=0, n=5}
  Soft Demodulation 4 : Subsystem  mask{w=3, f=0, n=4}
  Soft Demodulation 5 : Subsystem  mask{w=3, f=0, n=3}
  Soft Demodulation 6 : Subsystem  mask{w=3, f=0, n=2}
  Soft Demodulation 7 : Subsystem  mask{w=3, f=0, n=1}
  concat : hdlsllib/Logic and Bit Operations/Bit Concat  numInputs=8
  llr : Outport
  wires:
  valid/1 -> Soft Demodulation 0/1(valid), Soft Demodulation 1/1(valid), Soft Demodulation 2/1(valid), Soft Demodulation 3/1(valid), Soft Demodulation 4/1(valid), Soft Demodulation 5/1(valid), Soft Demodulation 6/1(valid), Soft Demodulation 7/1(valid)
  real/1 -> Soft Demodulation 0/2(real), Soft Demodulation 1/2(real), Soft Demodulation 2/2(real), Soft Demodulation 3/2(real), Soft Demodulation 4/2(real), Soft Demodulation 5/2(real), Soft Demodulation 6/2(real), Soft Demodulation 7/2(real)
  imag/1 -> Soft Demodulation 0/3(imag), Soft Demodulation 1/3(imag), Soft Demodulation 2/3(imag), Soft Demodulation 3/3(imag), Soft Demodulation 4/3(imag), Soft Demodulation 5/3(imag), Soft Demodulation 6/3(imag), Soft Demodulation 7/3(imag)
  scale/1 -> Soft Demodulation 0/4(LLR Scale), Soft Demodulation 1/4(LLR Scale), Soft Demodulation 2/4(LLR Scale), Soft Demodulation 3/4(LLR Scale), Soft Demodulation 4/4(LLR Scale), Soft Demodulation 5/4(LLR Scale), Soft Demodulation 6/4(LLR Scale), Soft Demodulation 7/4(LLR Scale)
  Soft Demodulation 0/1(LLR Values) -> concat/1
  Soft Demodulation 1/1(LLR Values) -> concat/2
  Soft Demodulation 2/1(LLR Values) -> concat/3
  Soft Demodulation 3/1(LLR Values) -> concat/4
  Soft Demodulation 4/1(LLR Values) -> concat/5
  Soft Demodulation 5/1(LLR Values) -> concat/6
  Soft Demodulation 6/1(LLR Values) -> concat/7
  Soft Demodulation 7/1(LLR Values) -> concat/8
  concat/1 -> llr/1

== system fec_ber_hw_V2/Soft Demodulation/Subsystem ==
  In1 : Inport
  Enable : EnablePort
  To Workspace : ToWorkspace  VariableName=llr_0  SampleTime=-1
      settings: Save2DSignal=2-D array (concatenate along first dimension)
  wires:
  In1/1 -> To Workspace/1

== system fec_ber_hw_V2/Soft Demodulation/byte_count ==
  reset : Inport
  en : Inport  Port=2
  Delay3 : Delay  DelayLength=1
  Delay5 : Delay  DelayLength=1
  HDL Counter1 : hdlsllib/Sources/HDL Counter  CountType=Count limited  CountInit=0  CountStep=1  CountMax=3  CountFromType=Initial value  CountFrom=0  CountResetPort=on  CountLoadPort=off  CountEnbPort=on  CountDirPort=off  CountDataType=Unsigned  CountWordLen=2  CountFracLen=0  CountSampTime=1
  OR : Logic  Operator=OR  IconShape=distinctive  AllPortsSameDT=off  OutDataTypeStr=boolean
  falling_edge : Subsystem
  tvalid hold : Subsystem
  count : Outport
  enable : Outport  Port=2
  wires:
  en/1 -> tvalid hold/1(en)
  OR/1 -> HDL Counter1/1
  reset/1 -> Delay3/1
  HDL Counter1/1 -> count/1
  Delay3/1 -> OR/1
  falling_edge/1(pulse) -> OR/2
  Delay5/1 -> enable/1, HDL Counter1/2, falling_edge/1(in)
  tvalid hold/1(" ") -> Delay5/1

== system fec_ber_hw_V2/Soft Demodulation/interface_creator ==
  data_in : Inport
  count : Inport  Port=2
  en : Inport  Port=3
  valid : Inport  Port=4
  AND{,1..2,4..7} (7 alike) : Logic  IconShape=distinctive  AllPortsSameDT=off  OutDataTypeStr=boolean
  Constant1 : Constant  Value=0  OutDataTypeStr=fixdt(0,96,0)  SampleTime=-1
  Constant2 : Constant  Value=0  OutDataTypeStr=fixdt(0,2,0)  SampleTime=-1
  Constant3 : Constant  OutDataTypeStr=fixdt(0,2,0)  SampleTime=-1
  Constant4 : Constant  Value=2  OutDataTypeStr=fixdt(0,2,0)  SampleTime=-1
  Constant5 : Constant  Value=3  OutDataTypeStr=fixdt(0,2,0)  SampleTime=-1
  Delay : Delay  DelayLength=1
  Delay1 : Delay  DelayLength=1
  Equal{,1..3} (4 alike) : RelationalOperator  Operator===  OutDataTypeStr=boolean  RndMeth=Simplest
  Multiport Switch : MultiPortSwitch  DataPortOrder=Zero-based contiguous  Inputs=2  zeroidx=on
  latch1 : Subsystem
  latch10 : Subsystem
  latch11 : Subsystem
  latch2 : Subsystem
  latch3 : Subsystem
  latch4 : Subsystem
  latch5 : Subsystem
  latch6 : Subsystem
  latch7 : Subsystem
  latch8 : Subsystem
  latch9 : Subsystem
  rising_edge : Subsystem
  tvalid hold : Subsystem
  tvalid hold1 : Subsystem
  tvalid hold2 : Subsystem
  tvalid hold3 : Subsystem
  lane_0_tvalid : Outport
  lane_0_tdata : Outport  Port=2
  lane_1_tvalid : Outport  Port=3
  lane_1_tdata : Outport  Port=4
  lane_2_tvalid : Outport  Port=5
  lane_2_tdata : Outport  Port=6
  lane_3_tvalid : Outport  Port=7
  lane_3_tdata : Outport  Port=8
  wires:
  AND/1 -> tvalid hold3/1(en)
  latch6/1(data_out) -> AND/2
  AND7/1 -> rising_edge/1(in), latch10/2(en), latch6/1(data)
  latch4/1(data_out) -> AND2/2
  Constant3/1 -> Equal1/2
  latch10/1(data_out) -> latch11/1(data_in)
  Equal/1 -> AND4/2
  Equal1/1 -> AND5/2
  latch5/1(data_out) -> AND1/2
  AND1/1 -> tvalid hold2/1(en)
  Equal2/1 -> AND6/2
  rising_edge/1(pulse) -> tvalid hold/1(en), AND2/1, AND1/1, AND/1, latch11/2(en), latch2/2(en), latch3/2(en), latch1/2(en)
  Constant2/1 -> Equal/2
  latch7/1(data_out) -> latch3/1(data_in)
  AND4/1 -> latch7/2(en), latch4/2(reset), latch5/2(reset), latch6/2(reset)
  latch9/1(data_out) -> latch2/1(data_in)
  en/1 -> AND4/1, AND7/1, AND6/1, AND5/1
  Constant5/1 -> Equal3/2
  Constant4/1 -> Equal2/2
  AND5/1 -> latch4/1(data), latch8/2(en)
  AND6/1 -> latch5/1(data), latch9/2(en)
  AND2/1 -> tvalid hold1/1(en)
  latch8/1(data_out) -> latch1/1(data_in)
  Multiport Switch/1 -> latch9/1(data_in), latch8/1(data_in), latch7/1(data_in), latch10/1(data_in)
  Equal3/1 -> AND7/2
  count/1 -> Equal/1, Equal1/1, Equal2/1, Equal3/1
  latch3/1(data_out) -> lane_0_tdata/1
  latch1/1(data_out) -> lane_1_tdata/1
  latch2/1(data_out) -> lane_2_tdata/1
  latch11/1(data_out) -> lane_3_tdata/1
  valid/1 -> Delay1/1
  data_in/1 -> Delay/1
  Constant1/1 -> Multiport Switch/2
  Delay/1 -> Multiport Switch/3
  Delay1/1 -> Multiport Switch/1
  tvalid hold/1(" ") -> lane_0_tvalid/1
  tvalid hold1/1(" ") -> lane_1_tvalid/1
  tvalid hold2/1(" ") -> lane_2_tvalid/1
  tvalid hold3/1(" ") -> lane_3_tvalid/1

== system fec_ber_hw_V2/Soft Demodulation1/SSR ==
  data_wide : Inport
  Bit Slice 0 : hdlsllib/Logic and Bit Operations/Bit Slice  lidx=2  ridx=0
      settings: SourceProductBaseCode=SL
  Bit Slice 1 : hdlsllib/Logic and Bit Operations/Bit Slice  lidx=5  ridx=3
      settings: SourceProductBaseCode=SL
  Bit Slice 10 : hdlsllib/Logic and Bit Operations/Bit Slice  lidx=32  ridx=30
      settings: SourceProductBaseCode=SL
  Bit Slice 11 : hdlsllib/Logic and Bit Operations/Bit Slice  lidx=35  ridx=33
      settings: SourceProductBaseCode=SL
  Bit Slice 12 : hdlsllib/Logic and Bit Operations/Bit Slice  lidx=38  ridx=36
      settings: SourceProductBaseCode=SL
  Bit Slice 13 : hdlsllib/Logic and Bit Operations/Bit Slice  lidx=41  ridx=39
      settings: SourceProductBaseCode=SL
  Bit Slice 14 : hdlsllib/Logic and Bit Operations/Bit Slice  lidx=44  ridx=42
      settings: SourceProductBaseCode=SL
  Bit Slice 15 : hdlsllib/Logic and Bit Operations/Bit Slice  lidx=47  ridx=45
      settings: SourceProductBaseCode=SL
  Bit Slice 2 : hdlsllib/Logic and Bit Operations/Bit Slice  lidx=8  ridx=6
      settings: SourceProductBaseCode=SL
  Bit Slice 3 : hdlsllib/Logic and Bit Operations/Bit Slice  lidx=11  ridx=9
      settings: SourceProductBaseCode=SL
  Bit Slice 4 : hdlsllib/Logic and Bit Operations/Bit Slice  lidx=14  ridx=12
      settings: SourceProductBaseCode=SL
  Bit Slice 5 : hdlsllib/Logic and Bit Operations/Bit Slice  lidx=17  ridx=15
      settings: SourceProductBaseCode=SL
  Bit Slice 6 : hdlsllib/Logic and Bit Operations/Bit Slice  lidx=20  ridx=18
      settings: SourceProductBaseCode=SL
  Bit Slice 7 : hdlsllib/Logic and Bit Operations/Bit Slice  lidx=23  ridx=21
      settings: SourceProductBaseCode=SL
  Bit Slice 8 : hdlsllib/Logic and Bit Operations/Bit Slice  lidx=26  ridx=24
      settings: SourceProductBaseCode=SL
  Bit Slice 9 : hdlsllib/Logic and Bit Operations/Bit Slice  lidx=29  ridx=27
      settings: SourceProductBaseCode=SL
  mux : Mux  Inputs=16
  data_ssr : Outport
  wires:
  data_wide/1 -> Bit Slice 0/1, Bit Slice 1/1, Bit Slice 2/1, Bit Slice 3/1, Bit Slice 4/1, Bit Slice 5/1, Bit Slice 6/1, Bit Slice 7/1, Bit Slice 8/1, Bit Slice 9/1, Bit Slice 10/1, Bit Slice 11/1, Bit Slice 12/1, Bit Slice 13/1, Bit Slice 14/1, Bit Slice 15/1
  Bit Slice 0/1 -> mux/1
  Bit Slice 1/1 -> mux/2
  Bit Slice 2/1 -> mux/3
  Bit Slice 3/1 -> mux/4
  Bit Slice 4/1 -> mux/5
  Bit Slice 5/1 -> mux/6
  Bit Slice 6/1 -> mux/7
  Bit Slice 7/1 -> mux/8
  Bit Slice 8/1 -> mux/9
  Bit Slice 9/1 -> mux/10
  Bit Slice 10/1 -> mux/11
  Bit Slice 11/1 -> mux/12
  Bit Slice 12/1 -> mux/13
  Bit Slice 13/1 -> mux/14
  Bit Slice 14/1 -> mux/15
  Bit Slice 15/1 -> mux/16
  mux/1 -> data_ssr/1

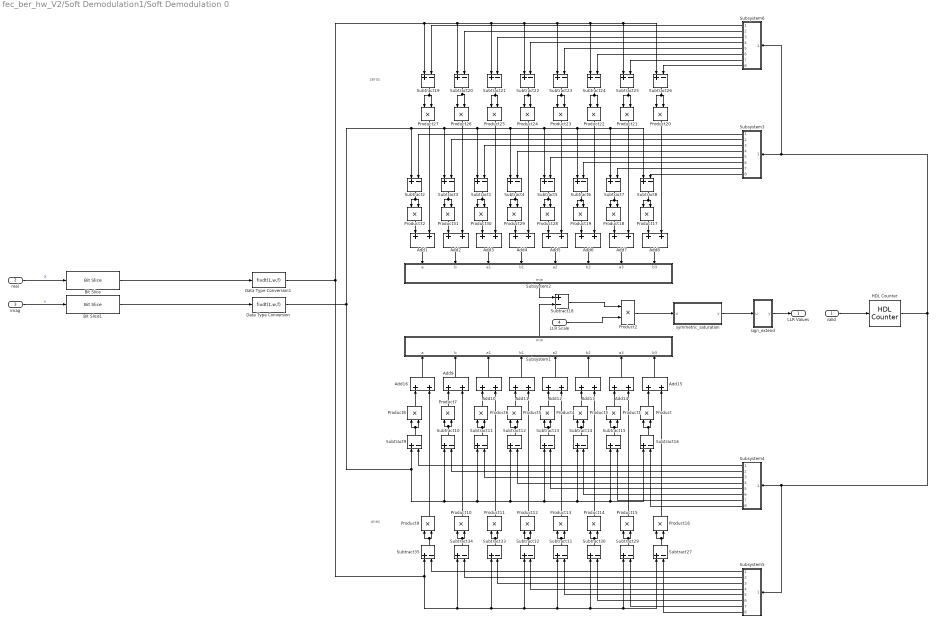
== system fec_ber_hw_V2/Soft Demodulation1/Soft Demodulation 0 ==
  note: zeros
  note: ones
  valid : Inport
  real : Inport  Port=2
  imag : Inport  Port=3
  LLR Scale : Inport  Port=4
  Add{1..16} (16 alike) : Sum  OutDataTypeStr=fixdt(1,(w+1)*2+1,f*2)  SaturateOnIntegerOverflow=on
  Bit Slice : hdlsllib/Logic and Bit Operations/Bit Slice  lidx=(n*w)-1  ridx=(n-1)*w
      settings: SourceProductBaseCode=SL
  Bit Slice1 : hdlsllib/Logic and Bit Operations/Bit Slice  lidx=(n*w)-1  ridx=(n-1)*w
      settings: SourceProductBaseCode=SL
  Data Type Conversion : DataTypeConversion  OutDataTypeStr=fixdt(1,w,f)  ConvertRealWorld=Stored Integer (SI)
  Data Type Conversion1 : DataTypeConversion  OutDataTypeStr=fixdt(1,w,f)  ConvertRealWorld=Stored Integer (SI)
  HDL Counter : hdlsllib/Sources/HDL Counter  CountType=Count limited  CountInit=0  CountStep=1  CountMax=3  CountFromType=Initial value  CountFrom=0  CountResetPort=off  CountLoadPort=off  CountEnbPort=on  CountDirPort=off  CountDataType=Unsigned  CountWordLen=2  CountFracLen=0  CountSampTime=1/(fs*2)
  Product{,1,3..16} (16 alike) : Product  SaturateOnIntegerOverflow=on
  Product{17..32} (16 alike) : Product
  Product2 : Product  RndMeth=Round  SaturateOnIntegerOverflow=on
  Subsystem1 : Subsystem
  Subsystem2 : Subsystem
  Subsystem3 : Subsystem
  Subsystem4 : Subsystem
  Subsystem5 : Subsystem
  Subsystem6 : Subsystem
  Subtract{1..16,19..27,29..35} (32 alike) : Sum  Inputs=+-  OutDataTypeStr=fixdt(1,w+1,f)  SaturateOnIntegerOverflow=on
  Subtract18 : Sum  Inputs=+-  OutDataTypeStr=fixdt(1,(w+1)*2+2,f*2)  SaturateOnIntegerOverflow=on
  sign_extend : Subsystem
  symmetric_saturation : MATLAB Function  TreatAsAtomicUnit=on
  LLR Values : Outport
  wires:
  Subsystem5/4(Out4) -> Subtract32/2
  Product6/1 -> Add10/1
  Product10/1 -> Add9/2
  Add12/1 -> Subsystem1/5(a2)
  Product1/1 -> Add14/1
  Subtract13/1 -> Product4/1, Product4/2
  Product/1 -> Add15/1
  Add1/1 -> Subsystem2/1(a)
  Product20/1 -> Add8/2
  Add3/1 -> Subsystem2/3(a1)
  Subsystem2/1(min) -> Subtract18/1
  Subsystem3/6(Out6) -> Subtract6/2
  Subtract10/1 -> Product7/2, Product7/1
  Subtract35/1 -> Product9/2, Product9/1
  real/1 -> Bit Slice/1  "X"
  Product25/1 -> Add3/2
  Product19/1 -> Add6/1
  Product3/1 -> Add13/1
  Add7/1 -> Subsystem2/7(a3)
  Product23/1 -> Add5/2
  Subtract21/1 -> Product25/1, Product25/2
  Product4/1 -> Add12/1
  LLR Scale/1 -> Product2/2
  Add10/1 -> Subsystem1/3(a1)
  Subtract24/1 -> Product22/1, Product22/2
  Subtract1/1 -> Product30/1, Product30/2
  Subsystem4/6(Out6) -> Subtract14/2
  Subtract18/1 -> Product2/1
  Product5/1 -> Add11/1
  Subsystem1/1(min) -> Subtract18/2
  Product22/1 -> Add6/2
  Subsystem3/2(Out2) -> Subtract3/2
  Add13/1 -> Subsystem1/6(b2)
  Product26/1 -> Add2/2
  Subtract19/1 -> Product27/1, Product27/2
  Product31/1 -> Add2/1
  Subsystem3/5(Out5) -> Subtract5/2
  Product30/1 -> Add3/1
  Add15/1 -> Subsystem1/8(b3)
  Product18/1 -> Add7/1
  Subtract4/1 -> Product29/2, Product29/1
  Subtract5/1 -> Product28/1, Product28/2
  Subtract2/1 -> Product32/1, Product32/2
  Add16/1 -> Subsystem1/1(a)
  imag/1 -> Bit Slice1/1  "y"
  Add14/1 -> Subsystem1/7(a3)
  Subtract23/1 -> Product23/2, Product23/1
  Subtract15/1 -> Product1/2, Product1/1
  Subtract9/1 -> Product8/2, Product8/1
  Subsystem3/1(Out1) -> Subtract2/2
  Product27/1 -> Add1/2
  Add8/1 -> Subsystem2/8(b3)
  Product14/1 -> Add13/2
  Product15/1 -> Add14/2
  Add2/1 -> Subsystem2/2(b)
  Add11/1 -> Subsystem1/4(b1)
  Add6/1 -> Subsystem2/6(b2)
  Subtract25/1 -> Product21/1, Product21/2
  Product21/1 -> Add7/2
  Subsystem3/4(Out4) -> Subtract4/2
  Subsystem4/5(Out5) -> Subtract13/2
  Product7/1 -> Add9/1
  Product8/1 -> Add16/1
  Product12/1 -> Add11/2
  Product28/1 -> Add5/1
  Subsystem3/3(Out3) -> Subtract1/2
  Subtract26/1 -> Product20/1, Product20/2
  Subsystem4/7(Out7) -> Subtract15/2
  Add9/1 -> Subsystem1/2(b)
  Product9/1 -> Add16/2
  Subsystem4/4(Out4) -> Subtract12/2
  Product17/1 -> Add8/1
  Subsystem4/3(Out3) -> Subtract11/2
  Subsystem5/2(Out2) -> Subtract34/2
  Subsystem5/3(Out3) -> Subtract33/2
  Product13/1 -> Add12/2
  Subtract3/1 -> Product31/1, Product31/2
  Product24/1 -> Add4/2
  Subsystem5/6(Out6) -> Subtract30/2
  Subsystem4/1(Out1) -> Subtract9/2
  Product16/1 -> Add15/2
  Subsystem3/7(Out7) -> Subtract7/2
  Subtract12/1 -> Product5/2, Product5/1
  Subsystem5/1(Out1) -> Subtract35/2
  Product32/1 -> Add1/1
  Subtract34/1 -> Product10/2, Product10/1
  Subtract11/1 -> Product6/2, Product6/1
  Subsystem5/7(Out7) -> Subtract29/2
  Subsystem5/8(Out8) -> Subtract27/2
  Subsystem4/2(Out2) -> Subtract10/2
  Subsystem4/8(Out8) -> Subtract16/2
  Product29/1 -> Add4/1
  Product11/1 -> Add10/2
  Add4/1 -> Subsystem2/4(b1)
  Subsystem3/8(Out8) -> Subtract8/2
  Add5/1 -> Subsystem2/5(a2)
  Subtract16/1 -> Product/2, Product/1
  Subsystem5/5(Out5) -> Subtract31/2
  Subtract14/1 -> Product3/1, Product3/2
  Subtract33/1 -> Product11/1, Product11/2
  Subtract32/1 -> Product12/1, Product12/2
  Subtract31/1 -> Product13/1, Product13/2
  Subtract30/1 -> Product14/1, Product14/2
  Subtract29/1 -> Product15/1, Product15/2
  Subtract27/1 -> Product16/1, Product16/2
  Subtract8/1 -> Product17/2, Product17/1
  Subtract7/1 -> Product18/1, Product18/2
  Subtract20/1 -> Product26/2, Product26/1
  Subtract22/1 -> Product24/1, Product24/2
  Subtract6/1 -> Product19/1, Product19/2
  Subsystem6/1(Out1) -> Subtract19/2
  Subsystem6/2(Out2) -> Subtract20/2
  Subsystem6/3(Out3) -> Subtract21/2
  Subsystem6/4(Out4) -> Subtract22/2
  Subsystem6/5(Out5) -> Subtract23/2
  Subsystem6/6(Out6) -> Subtract24/2
  Subsystem6/7(Out7) -> Subtract25/2
  Subsystem6/8(Out8) -> Subtract26/2
  valid/1 -> HDL Counter/1
  HDL Counter/1 -> Subsystem5/1(enb), Subsystem4/1(enb), Subsystem6/1(enb), Subsystem3/1(enb)
  symmetric_saturation/1(y) -> sign_extend/1(u)
  Product2/1 -> symmetric_saturation/1(u)
  sign_extend/1(y) -> LLR Values/1
  Data Type Conversion/1 -> Subtract2/1, Subtract3/1, Subtract1/1, Subtract4/1, Subtract5/1, Subtract6/1, Subtract8/1, Subtract7/1, Subtract9/1, Subtract10/1, Subtract11/1, Subtract12/1, Subtract13/1, Subtract14/1, Subtract16/1, Subtract15/1
  Data Type Conversion1/1 -> Subtract19/1, Subtract21/1, Subtract22/1, Subtract23/1, Subtract24/1, Subtract25/1, Subtract26/1, Subtract20/1, Subtract35/1, Subtract34/1, Subtract33/1, Subtract32/1, Subtract31/1, Subtract30/1, Subtract29/1, Subtract27/1
  Bit Slice1/1 -> Data Type Conversion/1
  Bit Slice/1 -> Data Type Conversion1/1
